simulink model "sim_logic_control"  (R2021b)
settings: Solver=VariableStepAuto  StartTime=0.0  StopTime=inf  RelTol=1e-3
libraries: flexy2_lib x1
settings Model: Creator=marekwadinger  LastModifiedBy=marekwadinger

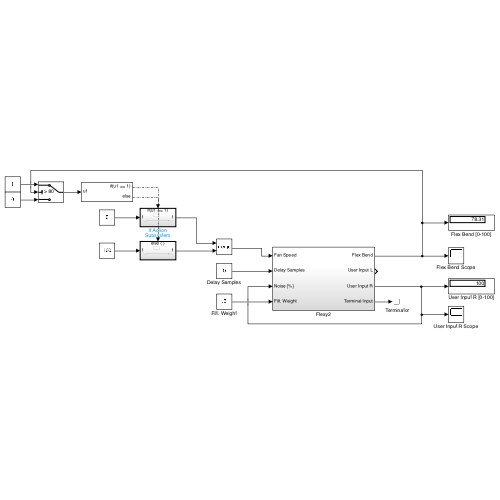
[thumbnail: Simulink's stored preview of the top-level diagram]
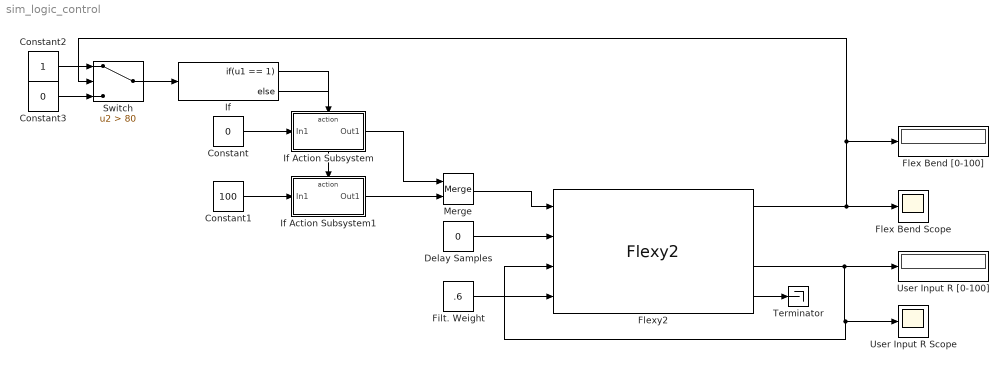
== system sim_logic_control ==
  Constant : Constant  Value=0
  Constant1 : Constant  Value=100
  Constant2 : Constant
  Constant3 : Constant  Value=0
  Delay Samples : Constant  Value=0
  Filt. Weight : Constant  Value=.6
  Flex Bend Scope : Scope
  Flex Bend [0-100] : Display
  Flexy2 : flexy2_lib/Flexy2  SystemSampleTime=-1  VariantActivationTime=update diagram  Latency=0  AutoFrameSizeCalculation=off
  If : If  IfExpression=u1 == 1
  If Action Subsystem : Subsystem  TreatAsAtomicUnit=on
  If Action Subsystem1 : Subsystem  TreatAsAtomicUnit=on
  Merge : Merge
  Switch : Switch  Criteria=u2 > Threshold  Threshold=80
  Terminator : Terminator
  User Input R Scope : Scope
  User Input R [0-100] : Display
  wires:
  Filt. Weight/1 -> Flexy2/4
  Flexy2/3 -> Flexy2/3, User Input R Scope/1, User Input R [0-100]/1
  Flexy2/1 -> Switch/2, Flex Bend [0-100]/1, Flex Bend Scope/1
  Flexy2/4 -> Terminator/1
  Delay Samples/1 -> Flexy2/2
  Merge/1 -> Flexy2/1
  If/1 -> If Action Subsystem/Action
  If/2 -> If Action Subsystem1/Action
  If Action Subsystem/1(Out1) -> Merge/1
  If Action Subsystem1/1(Out1) -> Merge/2
  Constant/1 -> If Action Subsystem/1(In1)
  Constant1/1 -> If Action Subsystem1/1(In1)
  Constant3/1 -> Switch/3
  Constant2/1 -> Switch/1
  Switch/1 -> If/1

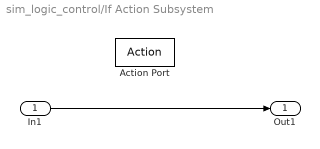
== system sim_logic_control/If Action Subsystem ==
  In1 : Inport
  Action Port : ActionPort  ActionPortLabel=if(u1 == 1)
  Out1 : Outport
  wires:
  In1/1 -> Out1/1

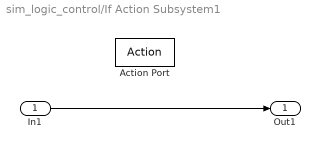
== system sim_logic_control/If Action Subsystem1 ==
  In1 : Inport
  Action Port : ActionPort  ActionPortLabel=else
  Out1 : Outport
  wires:
  In1/1 -> Out1/1
